simulink model "ServoControllerTaylor"  (R2021a)
settings: Solver=VariableStepAuto  StartTime=0.0  StopTime=20  RelTol=1e-3
values from neighbouring files (symbols this model uses):
  K = lqr(A,B,C_z'*Q_dfl*C_z,R)    [LQRCtrl.m]
undefined symbols (not defined in the file or in its folder): Cc_t, epsilon_0, eta_e0, F1_t, F2_t, p_0, T_0, v_0
settings Model: Creator=Sopagna  LastModifiedBy=sarmiento
settings SolverCC: AlgebraicLoopSolver=TrustRegion
settings DebuggingCC: SFMachineParentedDataDiag=warning

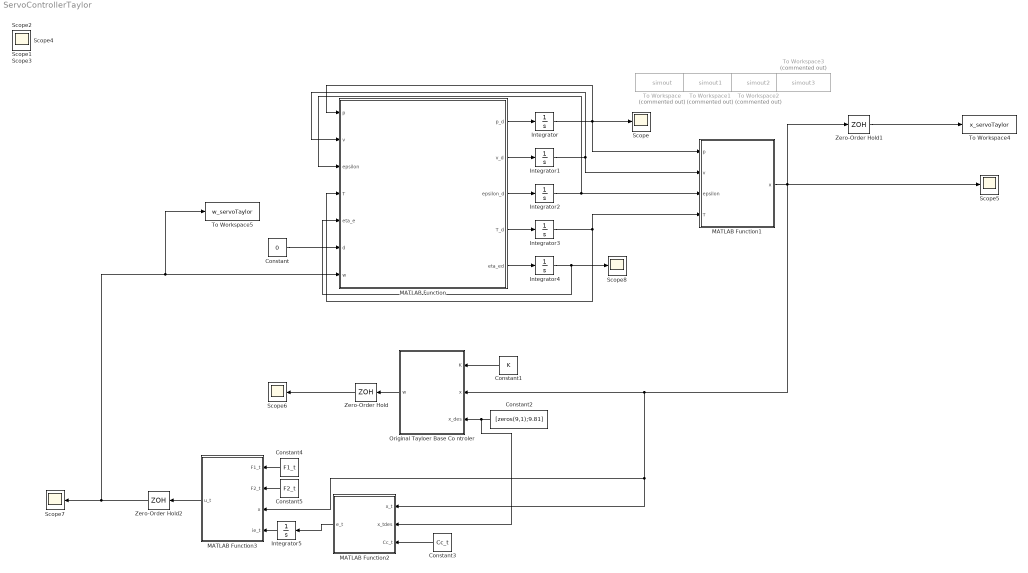
== system ServoControllerTaylor ==
  Constant : Constant  Value=0
  Constant1 : Constant  Value=K
  Constant2 : Constant  Value=[zeros(9,1);9.81]
  Constant3 : Constant  Value=Cc_t
  Constant4 : Constant  Value=F1_t
  Constant5 : Constant  Value=F2_t
  Integrator : Integrator  InitialCondition=p_0
  Integrator1 : Integrator  InitialCondition=v_0
  Integrator2 : Integrator  InitialCondition=epsilon_0
  Integrator3 : Integrator  InitialCondition=T_0
  Integrator4 : Integrator  InitialCondition=eta_e0
  Integrator5 : Integrator  InitialCondition=zeros(4,1)
  MATLAB Function : MATLAB Function  TreatAsAtomicUnit=on
  MATLAB Function1 : MATLAB Function  TreatAsAtomicUnit=on
  MATLAB Function2 : MATLAB Function  TreatAsAtomicUnit=on
  MATLAB Function3 : MATLAB Function  TreatAsAtomicUnit=on
  Original Tayloer Base Co ntroler : MATLAB Function  TreatAsAtomicUnit=on
  Scope{,1..8} (9 alike) : Scope
  To Workspace : ToWorkspace  Commented=on  VariableName=simout  SampleTime=-1
      settings: Save2DSignal=2-D array (concatenate along first dimension)
  To Workspace1 : ToWorkspace  Commented=on  VariableName=simout1  SampleTime=-1
      settings: Save2DSignal=2-D array (concatenate along first dimension)
  To Workspace2 : ToWorkspace  Commented=on  VariableName=simout2  SampleTime=-1
      settings: Save2DSignal=2-D array (concatenate along first dimension)
  To Workspace3 : ToWorkspace  Commented=on  VariableName=simout3  SampleTime=-1
      settings: Save2DSignal=2-D array (concatenate along first dimension)
  To Workspace4 : ToWorkspace  VariableName=x_servoTaylor  SampleTime=-1
      settings: Save2DSignal=2-D array (concatenate along first dimension)
  To Workspace5 : ToWorkspace  VariableName=w_servoTaylor  SampleTime=-1
      settings: Save2DSignal=2-D array (concatenate along first dimension)
  Zero-Order Hold : ZeroOrderHold  SampleTime=0.01
  Zero-Order Hold1 : ZeroOrderHold  SampleTime=0.01
  Zero-Order Hold2 : ZeroOrderHold  SampleTime=0.01
  wires:
  MATLAB Function/4(T_d) -> Integrator3/1
  MATLAB Function/3(epsilon_d) -> Integrator2/1
  MATLAB Function/2(v_d) -> Integrator1/1
  MATLAB Function/1(p_d) -> Integrator/1
  Integrator/1 -> MATLAB Function1/1(p), MATLAB Function/1(p), Scope/1
  Integrator1/1 -> MATLAB Function1/2(v), MATLAB Function/2(v)
  Integrator2/1 -> MATLAB Function1/3(epsilon), MATLAB Function/3(epsilon)
  Integrator3/1 -> MATLAB Function1/4(T), MATLAB Function/4(T)
  MATLAB Function/5(eta_ed) -> Integrator4/1
  Integrator4/1 -> Scope8/1, MATLAB Function/5(eta_e)
  Constant/1 -> MATLAB Function/6(d)
  Constant1/1 -> Original Tayloer Base Co ntroler/1(K)
  Constant2/1 -> MATLAB Function2/2(x_tdes), Original Tayloer Base Co ntroler/3(x_des)
  MATLAB Function1/1(x) -> Zero-Order Hold1/1, Scope5/1, MATLAB Function3/3(x), MATLAB Function2/1(x_t), Original Tayloer Base Co ntroler/2(x)
  Original Tayloer Base Co ntroler/1(w) -> Zero-Order Hold/1
  Constant3/1 -> MATLAB Function2/3(Cc_t)
  Integrator5/1 -> MATLAB Function3/4(ie_t)
  MATLAB Function2/1(e_t) -> Integrator5/1
  Constant4/1 -> MATLAB Function3/1(F1_t)
  Constant5/1 -> MATLAB Function3/2(F2_t)
  MATLAB Function3/1(u_t) -> Zero-Order Hold2/1
  Zero-Order Hold1/1 -> To Workspace4/1
  Zero-Order Hold/1 -> Scope6/1
  Zero-Order Hold2/1 -> To Workspace5/1, MATLAB Function/7(w), Scope7/1

== matlab function ServoControllerTaylor/Original Tayloer Base Co ntroler ==
  data: K input; w output; x input; x_des input
function w = fcn(K,x,x_des)

w = -K*(x-x_des);

== matlab function ServoControllerTaylor/MATLAB Function ==
  data: p input size=[3,1]; p_d output size=[3,1]; v input size=[3,1]; epsilon input size=[3,1]; T input size=1; eta_e input size=1; d input size=1; w input size=[4,1]; v_d output size=[3,1]; epsilon_d output size=[3,1]; T_d output size=1; eta_ed output size=1
function [p_d,v_d,epsilon_d,T_d,eta_ed] = fcn(p,v,epsilon,T,eta_e,d,w)
%==========================Input Variable================================
w1 = w(1:3); 
w2 = w(4); % Total Thrust
g = 9.81; % Gravity

%==========================Equation of Motion============================
p_d = v;    %Velocity
%Aerodynamic Damping Coefficient
K1 = 1;K2 = 1;K3 = 1; %Ns/m
F_aero = [K1*v(1);K2*v(2);K3*v(3)];
F_dis = [2.50;1.25;2];
v_d = r_z(epsilon,eta_e,d)*(T)+[0;0;-g]+F_dis; %Acceleration

%==========================First Way to get euler para derivative========
% epsilon_d = w1; %1st time derivative of euler parameters
% eta_e = sqrt(1-epsilon'*epsilon); % Angle of rotation

%==========================Second Way to get euler para derivative========
        K =0.5;
        euler = [epsilon;
         eta_e];
        C = euler.'*euler-1;
        J_E = J(euler);
        omega = 2*inv(J_E(1:3,:))*w1;
        e_d = 0.5*J_E*omega-K*C*euler;
epsilon_d = e_d(1:3);
eta_ed = e_d(4);

T_d = w2; %Time derivative of total thrust

% dx = [p_d;v_d;epsilon_d;T_d] +Dis;
% p_d = dx(1:3,:);
% v_d = dx(4:6,:);
% epsilon_d = dx(7:9,:);
% T_d = dx(10,:);

== matlab function ServoControllerTaylor/MATLAB Function1 ==
  data: p input; x output; v input; epsilon input; T input
function x = fcn(p,v,epsilon,T)

x = [p;
     v;
     epsilon;
     T];

== matlab function ServoControllerTaylor/MATLAB Function2 ==
  data: x_t input size=[10,1]; e_t output size=[4,1]; x_tdes input size=[10,1]; Cc_t input size=[4 10]
function e_t = fcn(x_t,x_tdes,Cc_t)
y = Cc_t*x_t;
yr = Cc_t*x_tdes;
e_t = (y-yr) ;

== matlab function ServoControllerTaylor/MATLAB Function3 ==
  data: F1_t input; u_t output; F2_t input; x input; ie_t input
function u_t = fcn(F1_t,F2_t,x,ie_t)

u_t = F1_t*x + F2_t*ie_t;
